simulink model "DUC_1"  (R2024b)
settings: Solver=FixedStepDiscrete  StartTime=0.0  StopTime=50000/fs_duc  FixedStep=1/fs_duc  RelTol=1e-3
values from neighbouring files (symbols this model uses):
  compFilt = design(compSpec,'SystemObject',true)    [main.m]
  fs_duc = fs_base*upsample_L    (= 6144000)    [main.m]
  hbFilt = design(hbSpec,'SystemObject',true)    [main.m]
  lowpassFilt = design(lowpassSpec,'SystemObject',true)    [main.m]
  N1_cycle = fix(up_L/2)    [duc_data_gen.m]    (also in main.m = 128)
  N2_cycle = fix(N1_cycle/2)    [duc_data_gen.m]    (also in main.m = 64)
  N3_cycle = 32    [main.m]
  N4_cycle = 16    [main.m]
libraries: dsphdlfiltering2 x3, hdlsllib x3, dsphdlsigops2 x2, dspmlti4 x1, simulink x1
settings Model: Creator=31651  LastModifiedBy=31651
settings OptimizationCC: BlockReduction=off  ConditionallyExecuteInputs=off
settings DebuggingCC: SignalRangeChecking=warning  SingleTaskRateTransMsg=error  ParamPrecisionLossAbsoluteDiffThreshold=0.0001  ParamPrecisionLossRelativeDiffThreshold=0.0001
settings RTWCC: GPUComputeCapability=3.5

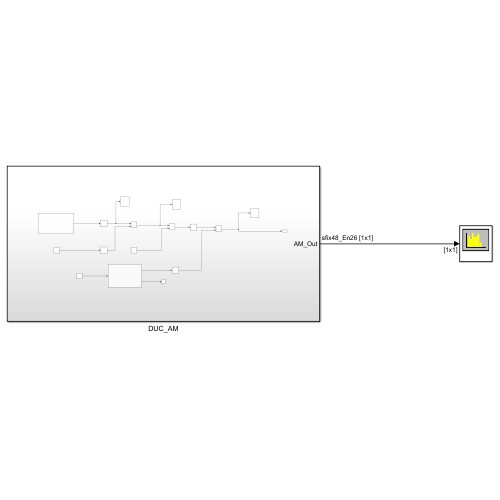
[thumbnail: Simulink's stored preview of the top-level diagram]
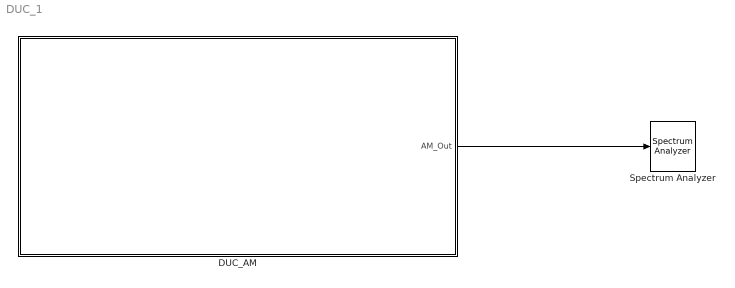
== system DUC_1 ==
  DUC_AM : Subsystem
  Spectrum Analyzer : SpectrumAnalyzer  WindowPosition=[229.000000,148.000000,800.000000,500.000000,]  Visible=on  ScopeFrameLocation=window  SpectrumType=RMS  Method=Welch  WindowInvariantSamplesPerUpdate=on  Span=6144000  StartFrequency=-3072000  StopFrequency=3072000  SpectrumUnits=Vrms  YLimits=[-0.06900745,0.62106946]  SelectedToolstripTab=spectrumAnalyzerToolstrip.estimationTab
  wires:
  DUC_AM/1(AM_Out) -> Spectrum Analyzer/1

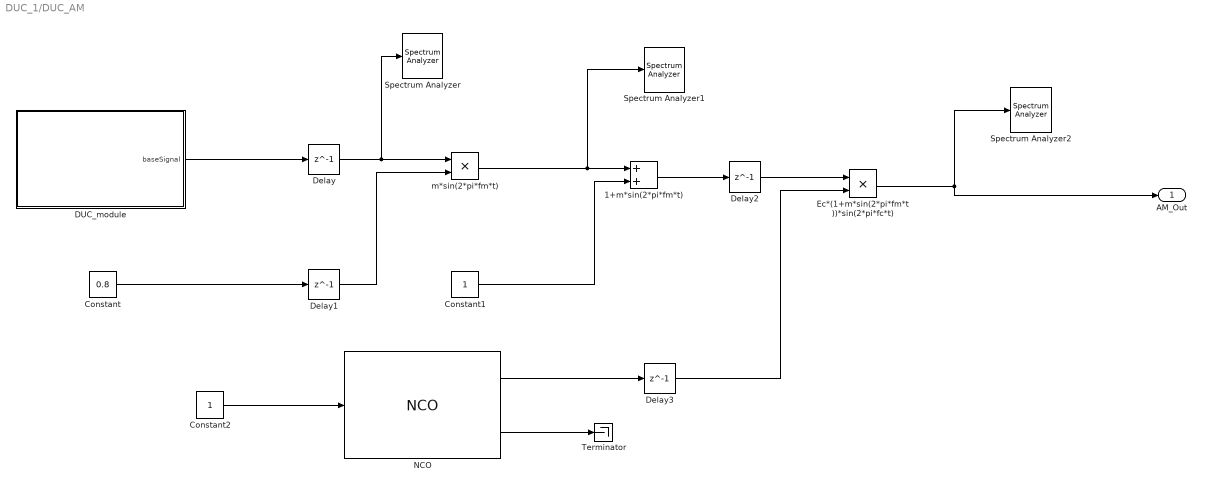
== system DUC_1/DUC_AM ==
  1+m*sin(2*pi*fm*t) : Sum
  Constant : Constant  Value=0.8  OutDataTypeStr=fixdt(1,16,15)  SampleTime=1/fs_duc
  Constant1 : Constant  OutDataTypeStr=int8  SampleTime=1/fs_duc
  Constant2 : Constant  OutDataTypeStr=boolean  SampleTime=1/fs_duc
  DUC_module : Subsystem
  Delay{,1..3} (4 alike) : Delay  DelayLength=1
  Ec*(1+m*sin(2*pi*fm*t))*sin(2*pi*fc*t) : Product
  NCO : dsphdlsigops2/NCO  PhaseIncrementSource=Property  PhaseIncrement=phInc  PhaseOffsetSource=Property  PhaseOffset=0  DitherSource=Property  NumDitherBits=ditherBits  SamplesPerFrame=1  LUTCompress=off  ResetAction=off  Waveform=Sine  PhasePort=off  SimulateUsing=Code generation  AccumulatorWL=Nnco  PhaseQuantization=on  NumQuantizerAccumulatorBits=Q  OutputDataType=Binary point scaling  OutputWL=16  OutputFL=2
      settings: LibrarySourceBlock=dsphdlsrcs2/NCO
  Spectrum Analyzer : SpectrumAnalyzer  WindowPosition=[277.000000,130.000000,891.000000,552.000000,]  Visible=on  ScopeFrameLocation=window  WindowInvariantSamplesPerUpdate=on  Span=6144000  StartFrequency=-3072000  StopFrequency=3072000  YLimits=[0.8408,110.2891]  ExpandToolstrip=on  SelectedToolstripTab=spectrumAnalyzerToolstrip.measurementsTab
  Spectrum Analyzer1 : SpectrumAnalyzer  WindowPosition=[368.000000,182.000000,800.000000,500.000000,]  Visible=on  ScopeFrameLocation=window  WindowInvariantSamplesPerUpdate=on  Span=6144000  StartFrequency=-3072000  StopFrequency=3072000  YLimits=[-18.78444079,90.57625682]
  Spectrum Analyzer2 : SpectrumAnalyzer  WindowPosition=[191.000000,581.000000,800.000000,500.000000,]  Visible=on  ScopeFrameLocation=window  WindowInvariantSamplesPerUpdate=on  Span=6144000  StartFrequency=-3072000  StopFrequency=3072000  YLimits=[-80.65848343,35.50867004]
  Terminator : Terminator
  m*sin(2*pi*fm*t) : Product
  AM_Out : Outport
  wires:
  NCO/1 -> Delay3/1
  NCO/2 -> Terminator/1
  DUC_module/1(baseSignal) -> Delay/1
  Constant1/1 -> 1+m*sin(2*pi*fm*t)/2
  1+m*sin(2*pi*fm*t)/1 -> Delay2/1
  m*sin(2*pi*fm*t)/1 -> 1+m*sin(2*pi*fm*t)/1, Spectrum Analyzer1/1
  Constant/1 -> Delay1/1
  Ec*(1+m*sin(2*pi*fm*t))*sin(2*pi*fc*t)/1 -> AM_Out/1, Spectrum Analyzer2/1
  Delay/1 -> m*sin(2*pi*fm*t)/1, Spectrum Analyzer/1
  Delay1/1 -> m*sin(2*pi*fm*t)/2
  Delay2/1 -> Ec*(1+m*sin(2*pi*fm*t))*sin(2*pi*fc*t)/1
  Delay3/1 -> Ec*(1+m*sin(2*pi*fm*t))*sin(2*pi*fc*t)/2
  Constant2/1 -> NCO/1

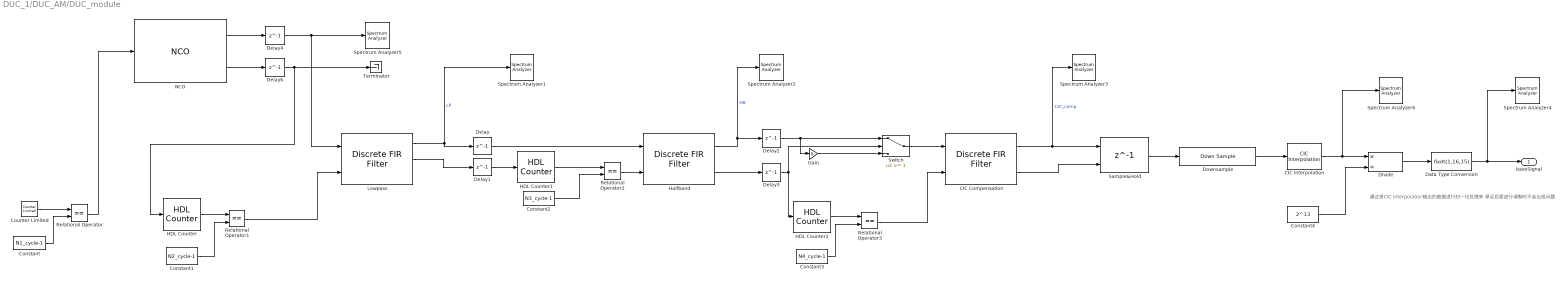
== system DUC_1/DUC_AM/DUC_module ==
  note: 通过将CIC interpolation输出的数据进行归一化处理来
      | 保证后面进行调制时不会出现问题
  CIC Interpolation : dspmlti4/CIC Interpolation  filtFrom=Dialog parameters  filtobj=Hm_interp  ftype=Interpolator  R=16  M=1  N=4  filterInternals=Minimum section word lengths  BPS=[16 16 16 16]  FLPS=0  outputWordLength=16  outputFracLength=0  launchFVT=off  framing=Allow multirate processing  OutputFrames=off
      settings: LibrarySourceBlock=|
      | dsphdlsupportfiltering/CIC
      | Interpolation
  CIC Compensation : dsphdlfiltering2/Discrete FIR Filter  NumeratorSource=Property  Numerator=compFilt.Numerator  NumeratorPrototype=[]  FilterStructure=Direct form systolic  SerializationOption=Minimum number of cycles between valid input samples  NumCycles=2  NumberOfMultipliers=2  SimulateUsing=Code generation  roundingMode=Floor  overflowMode=off  CoefficientsDataTypeStr=Inherit: Same word length as input  OutputDataTypeStr=fixdt(1,16,14)  ResetInputPort=off  HDLGlobalReset=off  CoeffMultiplier=Multiplier  UseMultForPow2Coeff=on
  Constant : Constant  Value=N1_cycle-1  OutDataTypeStr=uint8  SampleTime=1/fs_duc
  Constant1 : Constant  Value=N2_cycle-1  OutDataTypeStr=uint8  SampleTime=1/fs_duc
  Constant2 : Constant  Value=N3_cycle-1  OutDataTypeStr=uint8  SampleTime=1/fs_duc
  Constant3 : Constant  Value=N4_cycle-1  OutDataTypeStr=uint8  SampleTime=1/fs_duc
  Constant4 : Constant  Value=2^13  OutDataTypeStr=fixdt(1,16)  SampleTime=1/fs_duc
  Counter Limited : simulink/Sources/Counter Limited  uplimit=N1_cycle-1  tsamp=1/fs_duc
  Data Type Conversion : DataTypeConversion  OutDataTypeStr=fixdt(1,16,15)  SaturateOnIntegerOverflow=off  RndMeth=Floor
  Delay{,1..4,6} (6 alike) : Delay  DelayLength=1
  Divide : Product  Inputs=*/  OutDataTypeStr=fixdt(1,16,15)
  Downsample : DownSample  N=N4_cycle  RateOptions=Allow multirate processing
  Gain : Gain  Gain=0
  HDL Counter : hdlsllib/Sources/HDL Counter  CountType=Count limited  CountInit=0  CountStep=1  CountMax=N2_cycle-1  CountFromType=Initial value  CountFrom=0  CountResetPort=on  CountLoadPort=off  CountEnbPort=off  CountDirPort=off  CountHitOutputPort=off  CountDataType=Unsigned  CountWordLen=8  CountFracLen=0  CountSampTime=1
  HDL Counter1 : hdlsllib/Sources/HDL Counter  CountType=Count limited  CountInit=0  CountStep=1  CountMax=N3_cycle-1  CountFromType=Initial value  CountFrom=0  CountResetPort=on  CountLoadPort=off  CountEnbPort=off  CountDirPort=off  CountHitOutputPort=off  CountDataType=Unsigned  CountWordLen=8  CountFracLen=0  CountSampTime=1
  HDL Counter2 : hdlsllib/Sources/HDL Counter  CountType=Count limited  CountInit=0  CountStep=1  CountMax=N4_cycle-1  CountFromType=Initial value  CountFrom=0  CountResetPort=on  CountLoadPort=off  CountEnbPort=off  CountDirPort=off  CountHitOutputPort=off  CountDataType=Unsigned  CountWordLen=8  CountFracLen=0  CountSampTime=1
  Halfband : dsphdlfiltering2/Discrete FIR Filter  NumeratorSource=Property  Numerator=hbFilt.Numerator  NumeratorPrototype=[]  FilterStructure=Direct form systolic  SerializationOption=Minimum number of cycles between valid input samples  NumCycles=2  NumberOfMultipliers=2  SimulateUsing=Code generation  roundingMode=Floor  overflowMode=off  CoefficientsDataTypeStr=Inherit: Same word length as input  OutputDataTypeStr=fixdt(1,16,14)  ResetInputPort=off  HDLGlobalReset=off  CoeffMultiplier=Multiplier  UseMultForPow2Coeff=on
  Lowpass : dsphdlfiltering2/Discrete FIR Filter  NumeratorSource=Property  Numerator=lowpassFilt.Numerator  NumeratorPrototype=[]  FilterStructure=Partly serial systolic  SerializationOption=Maximum number of multipliers  NumCycles=2  NumberOfMultipliers=3  SimulateUsing=Code generation  roundingMode=Floor  overflowMode=off  CoefficientsDataTypeStr=Inherit: Same word length as input  OutputDataTypeStr=fixdt(1,16,14)  ResetInputPort=off  HDLGlobalReset=off  CoeffMultiplier=Multiplier  UseMultForPow2Coeff=on
  NCO : dsphdlsigops2/NCO  PhaseIncrementSource=Property  PhaseIncrement=phInc_b0  PhaseOffsetSource=Property  PhaseOffset=0  DitherSource=Property  NumDitherBits=ditherBits_base  SamplesPerFrame=1  LUTCompress=off  ResetAction=off  Waveform=Sine  PhasePort=off  SimulateUsing=Code generation  AccumulatorWL=Nnco_base  PhaseQuantization=on  NumQuantizerAccumulatorBits=Q_base  OutputDataType=Binary point scaling  OutputWL=16  OutputFL=14
      settings: LibrarySourceBlock=dsphdlsrcs2/NCO
  Relational Operator{,1..3} (4 alike) : RelationalOperator  Operator===  OutDataTypeStr=boolean  RndMeth=Simplest  InputSameDT=off
  Sample&Hold : Delay  DelayLength=1  ShowEnablePort=on  InputProcessing=Columns as channels (frame based)
      settings: InputPortMap=u0,e6
  Spectrum Analyzer1 : SpectrumAnalyzer  WindowPosition=[368.000000,182.000000,800.000000,500.000000,]  Visible=on  ScopeFrameLocation=window  WindowInvariantSamplesPerUpdate=on  Span=6144000  StartFrequency=-3072000  StopFrequency=3072000  YLimits=[-67.20448024,-2.96045691]
      settings: OpenAtSimulationStart=off
  Spectrum Analyzer2 : SpectrumAnalyzer  WindowPosition=[368.000000,173.000000,800.000000,519.000000,]  Visible=on  ScopeFrameLocation=window  WindowInvariantSamplesPerUpdate=on  Span=6144000  StartFrequency=-3072000  StopFrequency=3072000  YLimits=[-68.72958093,4.2771572]
      settings: OpenAtSimulationStart=off
  Spectrum Analyzer3 : SpectrumAnalyzer  WindowPosition=[368.000000,182.000000,800.000000,500.000000,]  Visible=on  ScopeFrameLocation=window  WindowInvariantSamplesPerUpdate=on  Span=6144000  StartFrequency=-3072000  StopFrequency=3072000  YLimits=[-70.11628299,11.42870347]
      settings: OpenAtSimulationStart=off
  Spectrum Analyzer4 : SpectrumAnalyzer  WindowPosition=[1322.000000,357.000000,800.000000,500.000000,]  ScopeFrameLocation=window  WindowInvariantSamplesPerUpdate=on  Span=6144000  StartFrequency=-3072000  StopFrequency=3072000  YLimits=[-12.25209277,14.36138924]
      settings: OpenAtSimulationStart=off
  Spectrum Analyzer5 : SpectrumAnalyzer  WindowPosition=[81.000000,354.000000,800.000000,500.000000,]  Visible=on  ScopeFrameLocation=window  WindowInvariantSamplesPerUpdate=on  Span=6144000  StartFrequency=-3072000  StopFrequency=3072000  YLimits=[-66.74735872,-9.86753031]
      settings: OpenAtSimulationStart=off
  Spectrum Analyzer6 : SpectrumAnalyzer  WindowPosition=[1322.000000,357.000000,800.000000,500.000000,]  Visible=on  ScopeFrameLocation=window  WindowInvariantSamplesPerUpdate=on  Span=6144000  StartFrequency=-3072000  StopFrequency=3072000  YLimits=[-6.575982758000009,110.79709645]
      settings: OpenAtSimulationStart=off
  Switch : Switch  Threshold=1  SaturateOnIntegerOverflow=off  InputSameDT=off
  Terminator : Terminator
  baseSignal : Outport
  wires:
  Counter Limited/1 -> Relational Operator/1
  Constant2/1 -> Relational Operator2/2
  HDL Counter/1 -> Relational Operator1/1
  Halfband/1 -> Delay2/1, Spectrum Analyzer2/1  "HB"
  Relational Operator/1 -> NCO/1
  Lowpass/1 -> Delay/1, Spectrum Analyzer1/1  "LP"
  Lowpass/2 -> Delay1/1
  Downsample/1 -> CIC Interpolation/1
  Constant1/1 -> Relational Operator1/2
  Constant3/1 -> Relational Operator3/2
  Constant/1 -> Relational Operator/2
  Switch/1 -> CIC Compensation/1
  Relational Operator3/1 -> CIC Compensation/2
  HDL Counter2/1 -> Relational Operator3/1
  CIC Compensation/1 -> Sample&Hold/1, Spectrum Analyzer3/1  "CIC_comp"
  HDL Counter1/1 -> Relational Operator2/1
  Halfband/2 -> Delay3/1
  Gain/1 -> Switch/3
  Sample&Hold/1 -> Downsample/1
  Relational Operator2/1 -> Halfband/2
  CIC Compensation/2 -> Sample&Hold/2
  NCO/1 -> Delay4/1
  NCO/2 -> Delay6/1
  Delay/1 -> Halfband/1
  Delay1/1 -> HDL Counter1/1
  Delay2/1 -> Gain/1, Switch/1
  Delay3/1 -> Switch/2, HDL Counter2/1
  Delay4/1 -> Lowpass/1, Spectrum Analyzer5/1
  Relational Operator1/1 -> Lowpass/2
  Delay6/1 -> HDL Counter/1, Terminator/1
  CIC Interpolation/1 -> Divide/1, Spectrum Analyzer6/1
  Data Type Conversion/1 -> Spectrum Analyzer4/1, baseSignal/1
  Divide/1 -> Data Type Conversion/1
  Constant4/1 -> Divide/2
